simulink model "LCK_old"  (R2018b)
settings: Solver=FixedStepDiscrete  StartTime=0.0  StopTime=inf  FixedStep=0.005  RelTol=1e-3
PostLoadFcn:
  | if any(exist('dsrtsu_mdlpostloadfcn', 'file') ~= 0), dsrtsu_mdlpostloadfcn('Execute', bdroot); end
values from neighbouring files (symbols this model uses):
  C_DEG2RAD = 0.0175    [LCK_Macro.sldd]
  C_KPH2MPS = 0.2778    [LCK_Macro.sldd]
  C_NEARZERO = 0.0001    [LCK_Macro.sldd]
  C_ONE = 1.0    [LCK_Macro.sldd]
  C_RAD2DEG = 57.2958    [LCK_Macro.sldd]
  C_ZERO = 0.0    [LCK_Macro.sldd]
  k_accel_pedal_pos_per_speed_x : value not decoded    [LCK_LogicPara.sldd]
  k_accel_pedal_pos_per_speed_z : value not decoded    [LCK_LogicPara.sldd]
  k_brake_suprress_hold = 1000.0    [LCK_LogicPara.sldd]
  k_driver_appl_torque_filt = 50.0    [LCK_LogicPara.sldd]
  k_driver_suppression_hold_time = 3000.0    [LCK_LogicPara.sldd]
  k_hands_on_wheel_hold_msec = 500.0    [LCK_LogicPara.sldd]
  k_hands_on_wheel_torque_hi = 0.2    [LCK_LogicPara.sldd]
  k_hands_on_wheel_torque_lo = 0.15    [LCK_LogicPara.sldd]
  k_handsoff_delay_cycles = 50.0    [LCK_LogicPara.sldd]
  k_handsoff_torq_Lo_CR = 0.3    [LCK_LogicPara.sldd]
  k_handson_delay_cycles = 5.0    [LCK_LogicPara.sldd]
  k_HighAccel_suppress_hold = 3000.0    [LCK_LogicPara.sldd]
  k_HLR_suprress_hold = 3000.0    [LCK_LogicPara.sldd]
  k_hs_StrAng_CR_threshold_z : value not decoded    [LCK_LogicPara.sldd]
  k_LC_Exit_Switch = 0.0    [LCK_LogicPara.sldd]
  k_LCG_Configured = 1.0    [LCK_LogicPara.sldd]
  k_LCK_A0_Rdy2Act_UseConst = 0.0    [LCK_LogicPara.sldd]
  k_LCK_A0Fac_ActSta : value not decoded    [LCK_CtrlPara.sldd]
  k_LCK_A0Fac_DrvStm : value not decoded    [LCK_CtrlPara.sldd]
  k_LCK_A0Shift_LftCurv : value not decoded    [LCK_CtrlPara.sldd]
  k_LCK_A0Shift_RgtCurv : value not decoded    [LCK_CtrlPara.sldd]
  k_LCK_A0Shift_StraLan = 0.0    [LCK_CtrlPara.sldd]
  k_LCK_A0ShiftFac_Dy_LftCurv : value not decoded    [LCK_CtrlPara.sldd]
  k_LCK_A0ShiftFac_Dy_RgtCurv : value not decoded    [LCK_CtrlPara.sldd]
  k_LCK_A0ShiftFac_Vspd : value not decoded    [LCK_CtrlPara.sldd]
  k_LCK_accel_inhibit_thold = 35.0    [LCK_LogicPara.sldd]
  k_LCK_Active2Ready_Mask = 255.0    [LCK_LogicPara.sldd]
  k_LCK_CvatRateBks : value not decoded    [LCK_CtrlPara.sldd]
  k_LCK_CvatrBks : value not decoded    [LCK_CtrlPara.sldd]
  k_LCK_DFac_Dy : value not decoded    [LCK_CtrlPara.sldd]
  k_LCK_DFac_Dy_Curv : value not decoded    [LCK_CtrlPara.sldd]
  k_LCK_DFac_HaCurCen : value not decoded    [LCK_CtrlPara.sldd]
  k_LCK_DFac_HaCurSid : value not decoded    [LCK_CtrlPara.sldd]
  k_LCK_DFac_HadCurCen : value not decoded    [LCK_CtrlPara.sldd]
  k_LCK_DFac_HadCurSid : value not decoded    [LCK_CtrlPara.sldd]
  k_LCK_DFac_HadStrCen : value not decoded    [LCK_CtrlPara.sldd]
  k_LCK_DFac_HadStrSid : value not decoded    [LCK_CtrlPara.sldd]
  k_LCK_DFac_HaStrCen : value not decoded    [LCK_CtrlPara.sldd]
  k_LCK_DFac_HaStrSid : value not decoded    [LCK_CtrlPara.sldd]
  k_LCK_DFac_Rad : value not decoded    [LCK_CtrlPara.sldd]
  k_LCK_DFac_SA_CurCen : value not decoded    [LCK_CtrlPara.sldd]
  k_LCK_DFac_SA_CurSid : value not decoded    [LCK_CtrlPara.sldd]
  k_LCK_DFac_SA_StrCen : value not decoded    [LCK_CtrlPara.sldd]
  k_LCK_DFac_SA_StrSid : value not decoded    [LCK_CtrlPara.sldd]
  k_LCK_DFac_SS_CurCen : value not decoded    [LCK_CtrlPara.sldd]
  k_LCK_DFac_SS_CurSid : value not decoded    [LCK_CtrlPara.sldd]
  k_LCK_DFac_SS_StrCen : value not decoded    [LCK_CtrlPara.sldd]
  k_LCK_DFac_SS_StrSid : value not decoded    [LCK_CtrlPara.sldd]
  k_LCK_DFac_Vspd : value not decoded    [LCK_CtrlPara.sldd]
  k_LCK_DlyTm_DrvStim = 0.2    [LCK_CtrlPara.sldd]
  k_LCK_DTermMax = 2.0    [LCK_CtrlPara.sldd]
  k_LCK_DyBks_Curv : value not decoded    [LCK_CtrlPara.sldd]
  k_LCK_Enable_POOnly = 1.0    [LCK_LogicPara.sldd]
  k_LCK_Entry_DistBuffer = 0.1    [LCK_LogicPara.sldd]
  k_LCK_Fac_Vspd2RngThr_FalRec = 0.23    [LCK_CtrlPara.sldd]
  k_LCK_Ffw_CvatSwh = 0.0    [LCK_CtrlPara.sldd]
  k_LCK_Ffw_DyBks : value not decoded    [LCK_CtrlPara.sldd]
  k_LCK_Ffw_TimCon_CmdFlt = 0.0    [LCK_CtrlPara.sldd]
  k_LCK_FfwDeltaFac_Rad_Lft : value not decoded    [LCK_CtrlPara.sldd]
  k_LCK_FfwDeltaFac_Rad_Rgt : value not decoded    [LCK_CtrlPara.sldd]
  k_LCK_FfwDeltaFac_Vspd : value not decoded    [LCK_CtrlPara.sldd]
  k_LCK_FfwFac_CvatRate_Lft : value not decoded    [LCK_CtrlPara.sldd]
  k_LCK_FfwFac_CvatRate_Rgt : value not decoded    [LCK_CtrlPara.sldd]
  k_LCK_FfwFac_Dy : value not decoded    [LCK_CtrlPara.sldd]
  k_LCK_FfwFac_Rad_Lft : value not decoded    [LCK_CtrlPara.sldd]
  k_LCK_FfwFac_Rad_Rgt : value not decoded    [LCK_CtrlPara.sldd]
  k_LCK_FfwFac_Vspd : value not decoded    [LCK_CtrlPara.sldd]
  k_LCK_FfwTorq_Cvat : value not decoded    [LCK_CtrlPara.sldd]
  k_LCK_HAFac_ActSta : value not decoded    [LCK_CtrlPara.sldd]
  k_LCK_HAFac_DrvStm : value not decoded    [LCK_CtrlPara.sldd]
  k_LCK_HaloTime = 2000.0    [LCK_LogicPara.sldd]
  k_LCK_HaloTime_Switch = 0.0    [LCK_LogicPara.sldd]
  k_LCK_HARFac_ActSta : value not decoded    [LCK_CtrlPara.sldd]
  k_LCK_HARFac_DrvStm : value not decoded    [LCK_CtrlPara.sldd]
  k_LCK_Hed_DyBks : value not decoded    [LCK_CtrlPara.sldd]
  k_LCK_HedAngDiffX : value not decoded    [LCK_CtrlPara.sldd]
  k_LCK_HedAngRateDiffX : value not decoded    [LCK_CtrlPara.sldd]
  k_LCK_HndsOnWhel_DlyTm_Idl2Rdy = 0.0    [LCK_LogicPara.sldd]
  k_LCK_host_veh_width = 1.86    [LCK_LogicPara.sldd]
  k_LCK_Idle2Ready_Mask = 239.0    [LCK_LogicPara.sldd]
  k_LCK_Junc_SusTime = 1.0    [LCK_LogicPara.sldd]
  k_LCK_KpKdDecSlopeLmt = 10.0    [LCK_CtrlPara.sldd]
  k_LCK_KpKdIncSlopeLmt = 5.0    [LCK_CtrlPara.sldd]
  k_LCK_Lat_Ctrl_DFac_Lft = 1.0    [LCK_CtrlPara.sldd]
  k_LCK_Lat_Ctrl_DFac_Rgt = 1.05    [LCK_CtrlPara.sldd]
  k_LCK_Lat_Ctrl_Kd = 0.8    [LCK_CtrlPara.sldd]
  k_LCK_Lat_Ctrl_Ki = 0.5    [LCK_CtrlPara.sldd]
  k_LCK_Lat_Ctrl_Kp = 0.7    [LCK_CtrlPara.sldd]
  k_LCK_Lat_Ctrl_Kp_NearGain = 0.7    [LCK_CtrlPara.sldd]
  k_LCK_Lat_Ctrl_PFac_Lft = 1.0    [LCK_CtrlPara.sldd]
  k_LCK_Lat_Ctrl_PFac_Rgt = 1.05    [LCK_CtrlPara.sldd]
  k_LCK_Lat_Ctrl_TimCon_CmdFlt = 5.0    [LCK_CtrlPara.sldd]
  k_LCK_Lat_DFac_Rad : value not decoded    [LCK_CtrlPara.sldd]
  k_LCK_Lat_DFac_SS_Cur : value not decoded    [LCK_CtrlPara.sldd]
  k_LCK_Lat_DFac_SS_Str : value not decoded    [LCK_CtrlPara.sldd]
  k_LCK_Lat_DFac_Vspd : value not decoded    [LCK_CtrlPara.sldd]
  k_LCK_Lat_DyBks : value not decoded    [LCK_CtrlPara.sldd]
  k_LCK_Lat_IFac_Rad : value not decoded    [LCK_CtrlPara.sldd]
  k_LCK_Lat_IFac_Vspd : value not decoded    [LCK_CtrlPara.sldd]
  k_LCK_Lat_ILmtFac_Dy_CurvLan : value not decoded    [LCK_CtrlPara.sldd]
  k_LCK_Lat_ILmtFac_Dy_StraLan : value not decoded    [LCK_CtrlPara.sldd]
  k_LCK_Lat_ILmtFac_Rad : value not decoded    [LCK_CtrlPara.sldd]
  k_LCK_Lat_ILmtFac_Rad_NearGain = 1.0    [LCK_CtrlPara.sldd]
  k_LCK_Lat_ILmtFac_Vspd_CurvLan : value not decoded    [LCK_CtrlPara.sldd]
  k_LCK_Lat_ILmtFac_Vspd_StraLan : value not decoded    [LCK_CtrlPara.sldd]
  k_LCK_Lat_ITermLmt_Dy = 1.0    [LCK_CtrlPara.sldd]
  k_LCK_Lat_KpKdDecSlopeLmt = 10.0    [LCK_CtrlPara.sldd]
  k_LCK_Lat_KpKdIncSlopeLmt = 10.0    [LCK_CtrlPara.sldd]
  k_LCK_Lat_PFac_Dy_InnLftCur : value not decoded    [LCK_CtrlPara.sldd]
  k_LCK_Lat_PFac_Dy_InnRgtCur : value not decoded    [LCK_CtrlPara.sldd]
  k_LCK_Lat_PFac_Dy_OutLftCur : value not decoded    [LCK_CtrlPara.sldd]
  k_LCK_Lat_PFac_Dy_OutRgtCur : value not decoded    [LCK_CtrlPara.sldd]
  k_LCK_Lat_PFac_Dy_Str : value not decoded    [LCK_CtrlPara.sldd]
  k_LCK_Lat_PFac_Rad : value not decoded    [LCK_CtrlPara.sldd]
  ... (+158 more)
undefined symbols (not defined in the file or in its folder): k_LCK_CurvBks, K_LCK_SPA0A1A2_LMRngCmp_y
libraries: LateralControl_fcns_lib x58, simulink x22
(part 16 of 45)

== system LCK_old/Lateral_Control_Module/Adas_Lateral_Control_LCK_Core/Module 11/Torque_Cmd_Rate_Limit ==
  TorqCmd : Inport  Description=_GWMH9P2.LKAFN.000_2_
  Lat_Ctrl_State : Inport  Port=2
  Vspd : Inport  Description=_GWMH9P2.LKAFN.000_2_  Port=3
  Abs : Abs
  Compare To Constant : simulink/Logic and Bit Operations/Compare To Constant  relop=>=  const=1  OutDataTypeStr=boolean
  Compare To Constant1 : simulink/Logic and Bit Operations/Compare To Constant  relop===  const=0  OutDataTypeStr=boolean
  Constant1 : Constant  Description=_GWMAB30P2.LCK.000_1301_  Value=0  OutDataTypeStr=single
  Constant2 : Constant  Description=_GWMAB30P2.LCK.000_1301_  Value=1500  OutDataTypeStr=single
  Constant3 : Constant  Description=_GWMAB30P2.LCK.000_1301_  OutDataTypeStr=single
  Gain : Gain  Description=_GWMH9P2.LKAFN.000_5_  Gain=ML_TIME_MSEC
  Gain1 : Gain  Description=_GWMH9P2.LKAFN.000_6_  Gain=ML_TIME_MSEC
  Gain2 : Gain  Description=_GWMH9P2.LKAFN.000_7_  Gain=-1
  Logical Operator : Logic  AllPortsSameDT=off  OutDataTypeStr=boolean
  Product1 : Product  Description=_GWMH9P2.LKAFN.000_8_  Inputs=**  InputSameDT=on  OutDataTypeStr=Inherit: Same as first input
  Product3 : Product  Description=_GWMH9P2.LKAFN.000_8_  Inputs=*/
  Product5 : Product  Description=_GWMH9P2.LKAFN.000_9_  Inputs=*/
  Relational Operator1 : RelationalOperator  Description=_GWMH9P2.LKAFN.000_11_  Operator=<  RndMeth=Nearest
  Relational Operator4 : RelationalOperator  Description=_GWMH9P2.LKAFN.000_12_  Operator=>  RndMeth=Nearest
  Sum : Sum  Description=_GWMH9P2.LKAFN.000_13_  Inputs=+-  InputSameDT=on  OutDataTypeStr=Inherit: Same as first input
  Sum1 : Sum  Description=_GWMH9P2.LKAFN.000_14_  OutDataTypeStr=Inherit: Same as first input
  Switch : Switch  Criteria=u2 > Threshold
  Switch19 : Switch  Description=_GWMH9P2.LKAFN.000_15_  Threshold=0.5  OutDataTypeStr=Inherit: Inherit via back propagation
  Switch20 : Switch  Description=_GWMH9P2.LKAFN.000_16_  Threshold=0.5  OutDataTypeStr=Inherit: Inherit via back propagation
  Switch4 : Switch  Description=_GWMAB30P2.LCK.000_1368_  Threshold=0.5
  Terminator : Terminator
  Trigger Hold Counter : LateralControl_fcns_lib/Trigger Hold Counter  SystemSampleTime=-1
  Unit Delay : UnitDelay  Description=_GWMH9P2.LKAFN.000_17_  SampleTime=-1
  Unit Delay1 : UnitDelay  Description=_GWMH9P2.LKAFN.000_17_  SampleTime=-1
  const : Constant  Description=_GWMH9P2.LKAFN.000_18_  Value=1000  OutDataTypeStr=single
  const1 : Constant  Description=_GWMH9P2.LKAFN.000_19_  Value=1000  OutDataTypeStr=single
  k_LCK_RatLmtFac_TorqCmd_Vspd : Lookup_n-D  NumberOfTableDimensions=1  BreakpointsForDimension1=k_LCK_VspdBks  IndexSearchMethod=Linear search  Table=k_LCK_RatLmtFac_TorqCmd_Vspd  ExtrapMethod=Clip  InternalRulePriority=Speed  RndMeth=Simplest  InputSameDT=on
  k_LCK_RatLmt_TorqCmd : Lookup_n-D  NumberOfTableDimensions=1  BreakpointsForDimension1=k_LCK_TorqCmdBks  IndexSearchMethod=Linear search  Table=k_LCK_RatLmt_TorqCmd  ExtrapMethod=Clip  InternalRulePriority=Speed  RndMeth=Simplest  InputSameDT=on
  TorqCmd_RateLimited : Outport  Description=_GWMH9P2.LKAFN.000_32_
  wires:
  Vspd/1 -> k_LCK_RatLmtFac_TorqCmd_Vspd/1
  k_LCK_RatLmtFac_TorqCmd_Vspd/1 -> Product1/1
  k_LCK_RatLmt_TorqCmd/1 -> Product1/2
  Sum/1 -> Switch19/3, Relational Operator1/2
  Product5/1 -> Switch19/1, Relational Operator1/1
  Gain/1 -> Product3/1
  Relational Operator4/1 -> Switch20/2
  Sum1/1 -> Unit Delay/1, TorqCmd_RateLimited/1
  Switch20/1 -> Sum1/1
  Unit Delay/1 -> Sum/2, Sum1/2
  Gain1/1 -> Product5/1
  const/1 -> Product3/2
  Gain2/1 -> Gain/1
  Relational Operator1/1 -> Switch19/2
  const1/1 -> Product5/2
  Product3/1 -> Relational Operator4/1, Switch20/1
  Switch19/1 -> Relational Operator4/2, Switch20/3
  Constant1/1 -> Switch4/3
  Compare To Constant/1 -> Logical Operator/1, Switch4/2
  TorqCmd/1 -> [TorqCmd], Switch4/1
  Switch4/1 -> Sum/1
  [TorqCmd] -> Abs/1
  Abs/1 -> k_LCK_RatLmt_TorqCmd/1
  Lat_Ctrl_State/1 -> Unit Delay1/1, Compare To Constant/1
  Unit Delay1/1 -> Compare To Constant1/1
  Compare To Constant1/1 -> Logical Operator/2
  Logical Operator/1 -> Trigger Hold Counter/1
  Constant2/1 -> Trigger Hold Counter/2
  Trigger Hold Counter/2 -> Terminator/1
  Trigger Hold Counter/1 -> [Init_Rate_Limit]
  Product1/1 -> Switch/3
  Switch/1 -> Gain1/1, Gain2/1
  [Init_Rate_Limit] -> Switch/2
  Constant3/1 -> Switch/1

== system LCK_old/Lateral_Control_Module/Adas_Lateral_Control_LCK_Core/Module 2/Calculation of Heading Angle Rate ==
  Yaw_Rate : Inport
  Road_Radius : Inport  Port=2
  Curvature_0 : Inport  Port=3
  Vspd : Inport  Port=4
  SPP_A0 : Inport  Port=5
  Str_Flag : Inport  Port=6
  Cur_Flag : Inport  Port=7
  " " : Constant  Tag={'output',{'name','$P','class','EXTERN_CAL','type','Float32'},'date',737503.54997206014}  Description=_GACA26P3.LCK.000_83_  Value=k_LCK_YawRateSign
  C_DEG2RAD : Gain  Gain=C_DEG2RAD
  C_KPH2MPS : Gain  Description=_GWMAB30P2.LCK.000_1299_  Gain=C_KPH2MPS
  C_RAD2DEG : Gain  Gain=C_RAD2DEG
  Constant2 : Constant  Description=_GWMAB30P3.LCK.000_155_  Value=0  OutDataTypeStr=single
  Gain1 : Gain  Gain=-1
  Product1 : Product  Description=_GWMAB30P2.LCK.000_1358_  RndMeth=Zero
  Product2 : Product  Description=_GWMAB30P2.LCK.000_1358_  Inputs=4  RndMeth=Zero
  Product8 : Product  Description=_GWMAB30P2.LCK.000_1358_  RndMeth=Zero
  Sign : Signum
  Sum1 : Sum  Description=_GWMAB30P2.LCK.000_1366_
  Sum4 : Sum  Description=_GWMAB30P2.LCK.000_1366_
  Switch1 : Switch  Criteria=u2 > Threshold
  Switch18 : Switch  Criteria=u2 > Threshold
  Switch4 : Switch  Description=_GWMAB30P2.LCK.000_1368_  Threshold=0.5
  k_LCK_YR_OffstFac_Dy_InnRgtCurv : Lookup_n-D  NumberOfTableDimensions=1  BreakpointsForDimension1=k_LCK_DyBks_Curv  BreakpointsForDimension2=K_LCK_SPA0A1A2_LMRngCmp_y  Table=k_LCK_YR_OffstFac_Dy_RgtCurv  ExtrapMethod=Clip  InternalRulePriority=Speed  RndMeth=Simplest  InputSameDT=on
  k_LCK_YR_OffstFac_Dy_LftCurv : Lookup_n-D  NumberOfTableDimensions=1  BreakpointsForDimension1=k_LCK_DyBks_Curv  BreakpointsForDimension2=K_LCK_SPA0A1A2_LMRngCmp_y  Table=k_LCK_YR_OffstFac_Dy_LftCurv  ExtrapMethod=Clip  InternalRulePriority=Speed  RndMeth=Simplest  InputSameDT=on
  k_LCK_YawRate_OffsetFac_Vspd : Lookup_n-D  NumberOfTableDimensions=1  BreakpointsForDimension1=k_LCK_VspdBks  IndexSearchMethod=Linear search  Table=k_LCK_YawRate_OffsetFac_Vspd  ExtrapMethod=Clip  InternalRulePriority=Speed  RndMeth=Simplest  InputSameDT=on
  k_LCK_YawRate_Offset_LftCurv : Lookup_n-D  NumberOfTableDimensions=1  BreakpointsForDimension1=k_LCK_RadBks  IndexSearchMethod=Linear search  Table=k_LCK_YawRate_Offset_LftCurv  ExtrapMethod=Clip  InternalRulePriority=Speed  RndMeth=Simplest  InputSameDT=on
  k_LCK_YawRate_Offset_RgtCurv : Lookup_n-D  NumberOfTableDimensions=1  BreakpointsForDimension1=k_LCK_RadBks  IndexSearchMethod=Linear search  Table=k_LCK_YawRate_Offset_RgtCurv  ExtrapMethod=Clip  InternalRulePriority=Speed  RndMeth=Simplest  InputSameDT=on
  Hed_Ang_Rat : Outport
  wires:
  C_DEG2RAD/1 -> Sum4/1
  Product8/1 -> Sum4/2
  C_RAD2DEG/1 -> Hed_Ang_Rat/1
  Sum1/1 -> C_DEG2RAD/1
  Sign/1 -> Gain1/1
  Sum4/1 -> C_RAD2DEG/1
  Road_Radius/1 -> k_LCK_YawRate_Offset_RgtCurv/1, k_LCK_YawRate_Offset_LftCurv/1
  Vspd/1 -> k_LCK_YawRate_OffsetFac_Vspd/1, C_KPH2MPS/1
  C_KPH2MPS/1 -> Product8/2
  Curvature_0/1 -> [Current_Curvature], Sign/1
  Str_Flag/1 -> Switch18/2
  Constant2/1 -> Switch18/1
  k_LCK_YawRate_Offset_LftCurv/1 -> Switch1/1
  k_LCK_YawRate_Offset_RgtCurv/1 -> Switch1/3
  Switch1/1 -> Switch18/3
  Gain1/1 -> Product2/1
  Switch18/1 -> Product2/2
  Product2/1 -> Sum1/2
  [Current_Curvature] -> Product8/1
  " "/1 -> Product1/2
  Yaw_Rate/1 -> Product1/1
  Product1/1 -> Sum1/1
  SPP_A0/1 -> k_LCK_YR_OffstFac_Dy_InnRgtCurv/1, k_LCK_YR_OffstFac_Dy_LftCurv/1
  k_LCK_YawRate_OffsetFac_Vspd/1 -> Product2/4
  Switch4/1 -> Product2/3
  Cur_Flag/1 -> Switch4/2, Switch1/2
  k_LCK_YR_OffstFac_Dy_LftCurv/1 -> Switch4/1
  k_LCK_YR_OffstFac_Dy_InnRgtCurv/1 -> Switch4/3

== system LCK_old/Lateral_Control_Module/Adas_Lateral_Control_LCK_Core/Module 3/Determination_Sig_Wekng_Factor ==
  A0Fac_ActSta : Inport
  HAFac_ActSta : Inport  Port=2
  HARFac_ActSta : Inport  Port=3
  A0Fac_DrvStm : Inport  Port=4
  HAFac_DrvStm : Inport  Port=5
  HARFac_DrvStm : Inport  Port=6
  Bus Creator4 : BusCreator  Inputs=3
  MinMax : MinMax  Inputs=2
  MinMax1 : MinMax  Inputs=2
  MinMax2 : MinMax  Inputs=2
  Sig_Wekng_Factor : Outport
  wires:
  A0Fac_ActSta/1 -> MinMax/1
  HAFac_DrvStm/1 -> MinMax1/2
  HAFac_ActSta/1 -> MinMax1/1
  Bus Creator4/1 -> Sig_Wekng_Factor/1
  MinMax/1 -> Bus Creator4/1  "A0_Wekng_Fac"
  MinMax2/1 -> Bus Creator4/3  "HAR_Wekng_Fac"
  MinMax1/1 -> Bus Creator4/2  "HA_Wekng_Fac"
  A0Fac_DrvStm/1 -> MinMax/2
  HARFac_ActSta/1 -> MinMax2/1
  HARFac_DrvStm/1 -> MinMax2/2
